simulink model "cxfpid_part3_ga_ant"  (Simulink 7.6)
settings: Solver=ode15s  StartTime=0.0  StopTime=100  RelTol=1e-3
PreLoadFcn:
  | L=1; M=1;
undefined symbols (not defined in the file or in its folder): Kd1, Kd2, Ki1, Ki2, Kp1, Kp2, L1, L2, M1, M2
settings Model: Creator=Professor Dingyu Xue  LastModifiedBy=Pragya
settings OptimizationCC: InitFltsAndDblsToZero=on
settings DebuggingCC: SolverPrmCheckMsg=none  StrictBusMsg=Warning

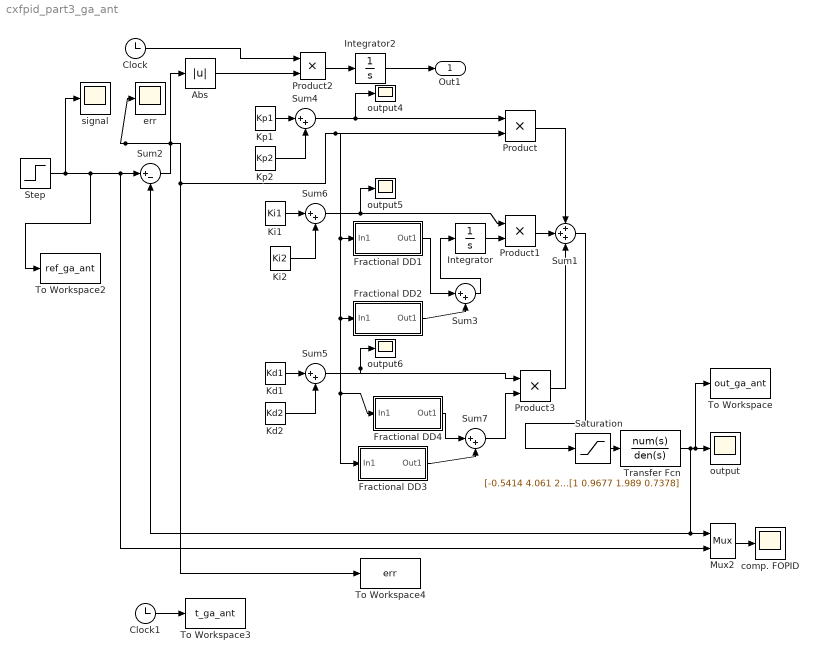
== system cxfpid_part3_ga_ant ==
  Abs : Abs
  Clock : Clock
      settings: Decimation=10
  Clock1 : Clock
      settings: Decimation=10
  Fractional DD1 : Subsystem  mask{gam=L1, ww=[1e-3 1e3], n=2, key=Modified Oustaloup's filter}
      mask prompts: gam "Derivative order gamma"; ww "Frequency range [wb,wh]"; n "Apprixmation order"; key "Selected filter"
      mask help: Fractional-order differentiator with Oustaloup's or modified Oustaloup's filter. The fitting frequency range and order should also be specified.
      mask init:
      | wb=ww(1); wh=ww(2); 
      | if key==1, G=ousta_fod(gam,n,wb,wh);
      | else, G=tf(new_fod(gam,n,wb,wh)); end
      | num=G.num{1}; den=G.den{1}; T=1/wh; str='Fractional\n';
      | if isnumeric(gam)
      | 	if gam>0, str=[str, 'Der  s^' num2str(0.01*round(100*gam)) ];
      | 	else, str=[str, 'Int  s^{' num2str(0.01*round(100*gam)) '}']; end
      | else, str=[str, 'Der  s^gam']; end
      mask StyleString: edit,edit,edit,popup(Oustaloup's filter|Modified Oustaloup's filter )
      mask Display: disp(str)
  Fractional DD2 : Subsystem  mask{gam=L2, ww=[1e-3 1e3], n=2, key=Modified Oustaloup's filter}
      mask prompts: gam "Derivative order gamma"; ww "Frequency range [wb,wh]"; n "Apprixmation order"; key "Selected filter"
      mask help: Fractional-order differentiator with Oustaloup's or modified Oustaloup's filter. The fitting frequency range and order should also be specified.
      mask init: same as cxfpid_part3_ga_ant/Fractional DD1
      mask StyleString: edit,edit,edit,popup(Oustaloup's filter|Modified Oustaloup's filter )
      mask Display: disp(str)
  Fractional DD3 : Subsystem  mask{gam=M2, ww=[1e-3 1e3], n=2, key=Modified Oustaloup's filter}
      mask prompts: gam "Derivative order gamma"; ww "Frequency range [wb,wh]"; n "Apprixmation order"; key "Selected filter"
      mask help: Fractional-order differentiator with Oustaloup's or modified Oustaloup's filter. The fitting frequency range and order should also be specified.
      mask init: same as cxfpid_part3_ga_ant/Fractional DD1
      mask StyleString: edit,edit,edit,popup(Oustaloup's filter|Modified Oustaloup's filter )
      mask Display: disp(str)
  Fractional DD4 : Subsystem  mask{gam=M1, ww=[1e-3 1e3], n=2, key=Modified Oustaloup's filter}
      mask prompts: gam "Derivative order gamma"; ww "Frequency range [wb,wh]"; n "Apprixmation order"; key "Selected filter"
      mask help: Fractional-order differentiator with Oustaloup's or modified Oustaloup's filter. The fitting frequency range and order should also be specified.
      mask init: same as cxfpid_part3_ga_ant/Fractional DD1
      mask StyleString: edit,edit,edit,popup(Oustaloup's filter|Modified Oustaloup's filter )
      mask Display: disp(str)
  Integrator : Integrator
  Integrator2 : Integrator
  Kd1 : Constant  Value=Kd1
  Kd2 : Constant  Value=Kd2
  Ki1 : Constant  Value=Ki1
  Ki2 : Constant  Value=Ki2
  Kp1 : Constant  Value=Kp1
  Kp2 : Constant  Value=Kp2
  Mux2 : Mux  Inputs=2
  Product{,1..3} (4 alike) : Product  RndMeth=Zero
  Saturation : Saturate  UpperLimit=2  LowerLimit=-2
  Step : Step  Time=0  SampleTime=0
  Sum1 : Sum  Inputs=+++
  Sum2 : Sum  Inputs=|+-
  Sum{3..7} (5 alike) : Sum  Inputs=|++
  To Workspace : ToWorkspace  VariableName=out_ga_ant  SampleTime=-1  SaveFormat=Array
  To Workspace2 : ToWorkspace  VariableName=ref_ga_ant  SampleTime=-1  SaveFormat=Array
  To Workspace3 : ToWorkspace  VariableName=t_ga_ant  SampleTime=-1  SaveFormat=Array
  To Workspace4 : ToWorkspace  VariableName=err  SampleTime=-1  SaveFormat=Array
  Transfer Fcn : TransferFcn  Numerator=[-0.5414 4.061 2.945]  Denominator=[1 0.9677 1.989 0.7378]
  comp. FOPID : Scope
      settings: TickLabels=on  TimeRange=10  YMin=0  YMax=2.1  SaveName=dc_pid1  DataFormat=Array
  err : Scope
      settings: TimeRange=15  YMin=1.23519  YMax=1.36521  SaveName=yy1  DataFormat=Array
  output{,4..6} (4 alike) : Scope
      output settings: TickLabels=on  TimeRange=10  YMin=0.25  YMax=1.75  SaveName=fopid  DataFormat=Array
      output4 settings: TickLabels=on  TimeRange=100  YMin=0.04  YMax=0.15  SaveName=outputdc  DataFormat=Array
      output5 settings: TickLabels=on  TimeRange=100  YMin=0.04  YMax=0.15  SaveName=outputdc1  DataFormat=Array
      output6 settings: TickLabels=on  TimeRange=100  YMin=0.04  YMax=0.15  SaveName=outputdc2  DataFormat=Array
  signal : Scope
      settings: TickLabels=on  TimeRange=100  YMin=1.23519  YMax=1.36521  SaveName=sig  DataFormat=Array
  Out1 : Outport
  wires:
  Sum2/1 -> err/1, To Workspace4/1, Product/2, Fractional DD1/1(In1), Fractional DD2/1(In1), Fractional DD4/1(In1), Fractional DD3/1(In1), Abs/1
  Transfer Fcn/1 -> Sum2/2, Mux2/1, output/1, To Workspace/1
  Mux2/1 -> comp. FOPID/1
  Integrator2/1 -> Out1/1
  Abs/1 -> Product2/2
  Clock/1 -> Product2/1
  Product2/1 -> Integrator2/1
  Step/1 -> signal/1, Sum2/1, Mux2/2, To Workspace2/1
  Saturation/1 -> Transfer Fcn/1
  Clock1/1 -> To Workspace3/1
  Kp1/1 -> Sum4/1
  Kd1/1 -> Sum5/1
  Sum4/1 -> output4/1, Product/1
  Sum6/1 -> output5/1, Product1/1
  Sum5/1 -> output6/1, Product3/1
  Product/1 -> Sum1/1
  Product1/1 -> Sum1/2
  Product3/1 -> Sum1/3
  Integrator/1 -> Product1/2
  Sum1/1 -> Saturation/1
  Kp2/1 -> Sum4/2
  Ki2/1 -> Sum6/2
  Kd2/1 -> Sum5/2
  Fractional DD2/1(Out1) -> Sum3/2
  Sum7/1 -> Product3/2
  Sum3/1 -> Integrator/1
  Fractional DD4/1(Out1) -> Sum7/1
  Fractional DD3/1(Out1) -> Sum7/2
  Ki1/1 -> Sum6/1
  Fractional DD1/1(Out1) -> Sum3/1

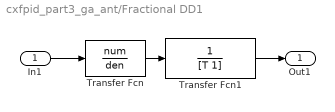
== system cxfpid_part3_ga_ant/Fractional DD1 ==
  In1 : Inport
  Transfer Fcn : TransferFcn  Numerator=num  Denominator=den
  Transfer Fcn1 : TransferFcn  Numerator=1  Denominator=[T 1]
  Out1 : Outport
  wires:
  Transfer Fcn1/1 -> Out1/1
  Transfer Fcn/1 -> Transfer Fcn1/1
  In1/1 -> Transfer Fcn/1

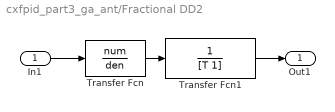
== system cxfpid_part3_ga_ant/Fractional DD2 ==
  In1 : Inport
  Transfer Fcn : TransferFcn  Numerator=num  Denominator=den
  Transfer Fcn1 : TransferFcn  Numerator=1  Denominator=[T 1]
  Out1 : Outport
  wires:
  Transfer Fcn1/1 -> Out1/1
  Transfer Fcn/1 -> Transfer Fcn1/1
  In1/1 -> Transfer Fcn/1

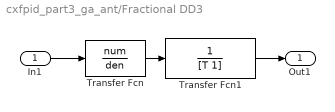
== system cxfpid_part3_ga_ant/Fractional DD3 ==
  In1 : Inport
  Transfer Fcn : TransferFcn  Numerator=num  Denominator=den
  Transfer Fcn1 : TransferFcn  Numerator=1  Denominator=[T 1]
  Out1 : Outport
  wires:
  Transfer Fcn1/1 -> Out1/1
  Transfer Fcn/1 -> Transfer Fcn1/1
  In1/1 -> Transfer Fcn/1

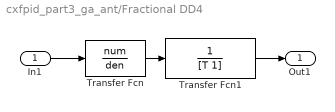
== system cxfpid_part3_ga_ant/Fractional DD4 ==
  In1 : Inport
  Transfer Fcn : TransferFcn  Numerator=num  Denominator=den
  Transfer Fcn1 : TransferFcn  Numerator=1  Denominator=[T 1]
  Out1 : Outport
  wires:
  Transfer Fcn1/1 -> Out1/1
  Transfer Fcn/1 -> Transfer Fcn1/1
  In1/1 -> Transfer Fcn/1
